simulink library "Weather_from_File_string"  (R2016b)
settings: Solver=ode45  StartTime=0.0  StopTime=10.0  RelTol=1e-3  EnableMultiTasking=on
undefined symbols (not defined in the file): t_sample
libraries: carnot x1
settings Model: Creator=lena.frank  LastModifiedBy=drhf
settings DataIOCC: LimitDataPoints=on  SaveFormat=Array  SignalLoggingSaveFormat=ModelDataLogs
settings OptimizationCC: ExpressionDepthLimit=2147483647  LifeSpan=inf
settings DebuggingCC: UnderspecifiedInitializationDetection=Classic  MergeDetectMultiDrivingBlocksExec=none  SolverPrmCheckMsg=warning  FcnCallInpInsideContextMsg=warning  StateNameClashWarn=warning  SFUnexpectedBacktrackingDiag=warning  SFNoUnconditionalDefaultTransitionDiag=warning  SFExecutionAtInitializationDiag=none
settings HardwareCC: ProdBitPerPointer=32  ProdBitPerSizeT=32  ProdBitPerPtrDiffT=32  ProdLargestAtomicFloat=None  ProdIntDivRoundTo=Undefined  ProdEndianess=Unspecified  ProdWordSize=32  ProdHWDeviceType=32-bit Generic
settings ModelReferenceCC: PropagateSignalLabelsOutOfModel=off
settings GRTTargetCC: TargetLangStandard=C89/C90 (ANSI)  GeneratePreprocessorConditionals=Disable all  CombineOutputUpdateFcns=off  GRTInterface=on
settings ConfigComp: CovMetricSettings=dw  CovHtmlReporting=on  CovSaveCumulativeToWorkspaceVar=on  CovSaveSingleToWorkspaceVar=on  CovExternalEMLEnable=off

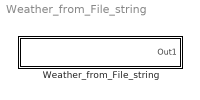
== system Weather_from_File_string ==
  Weather_from_File_string : Subsystem  mask(weather from file){file='DE_TRY2010_04_averageYear', ext=.mat}
      mask prompts: file "Name of file"; ext "Extension of file"
      mask help:
      | Input block for external weather data files. The file is read to the workspace. A "From Workspace" Block is used in the subsystem.
      | A Unit-Delay with the timestep of the weather data forces the model to a maximum timestep equal to the data acquisiton timestep.
      | Remark: Be carefull when using the TRY Data 2010 for Germany. The files are public and can be found in the parameter_set folder of this block. But there are bugs is the solar radiation data.
      mask init:
      | parampath = fullfile('Weather','Weather_from_File','parameter_set');
      | CarnotCallbacks_GetFiles;
      | warning('Weather_from_File_String is obsolete. Consider to replace it with Weather_Datafile.')
      mask Help: web(fullfile(path_carnot('help'),'weather_from_file.html'),'-helpbrowser')
      mask TypeOptions ext: .dat | .txt | .mat
      mask Display: disp(file)

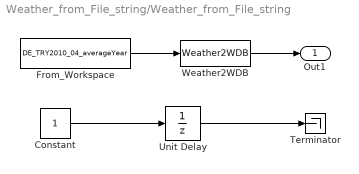
== system Weather_from_File_string/Weather_from_File_string ==
  Constant : Constant
  From_Workspace : FromWorkspace  VariableName=DE_TRY2010_04_averageYear  SampleTime=0  OutputAfterFinalValue=Setting to zero
  Terminator : Terminator
  Unit Delay : UnitDelay  SampleTime=t_sample
  Weather2WDB : carnot/Toolbox/Weather2WDB
  Out1 : Outport
  wires:
  From_Workspace/1 -> Weather2WDB/1
  Constant/1 -> Unit Delay/1
  Unit Delay/1 -> Terminator/1
  Weather2WDB/1 -> Out1/1
